simulink model "HANcoder_E407_GTSync_v4"  (R2018b)
settings: Solver=FixedStepDiscrete  StartTime=0.0  StopTime=1  FixedStep=0.01  RelTol=1e-3
PreLoadFcn:
  | librarySetup
  | eval([bdroot,'_startup']) %Calling [modelName]_startup.m
values from neighbouring files (symbols this model uses):
  basic_cycle_duration = TM12 + COMP_duration    (= 495)    [HANcoder_E407_GTSync_v4_startup.m]
  COM_Period = 100    [HANcoder_E407_GTSync_v4_startup.m]
  COM_Phase = COM_Period/2    (= 50)    [HANcoder_E407_GTSync_v4_startup.m]
  comm_delay_estimation = 20    [HANcoder_E407_GTSync_v4_startup.m]
  frequency_IRQ = 20    [HANcoder_E407_GTSync_v4_startup.m]
  HANtuneOverride = Simulink.Parameter    [HANcoder_E407_GTSync_v4_startup.m]
  idle_time_init = basic_cycle_duration*matrix_rows    (= 990)    [HANcoder_E407_GTSync_v4_startup.m]
  LED_ticks_toggle = 10000    [HANcoder_E407_GTSync_v4_startup.m]
  Master_Role = 1    [HANcoder_E407_GTSync_v4_startup.m]
  matrix_rows = 2    [HANcoder_E407_GTSync_v4_startup.m]
  Slave_Role = 2    [HANcoder_E407_GTSync_v4_startup.m]
  Sync_ID = 1    [HANcoder_E407_GTSync_v4_startup.m]
  time_difference_threshold = 500    [HANcoder_E407_GTSync_v4_startup.m]
  TM0 = basic_cycle_start    (= 5)    [HANcoder_E407_GTSync_v4_startup.m]
  TM1 = TM0 + COMM_duration    (= 105)    [HANcoder_E407_GTSync_v4_startup.m]
  TM10 = TM9  + COMP_duration    (= 465)    [HANcoder_E407_GTSync_v4_startup.m]
  TM11 = TM10 + COMP_duration    (= 475)    [HANcoder_E407_GTSync_v4_startup.m]
  TM12 = TM11 + COMP_duration    (= 485)    [HANcoder_E407_GTSync_v4_startup.m]
  TM2 = TM1 + COMP_duration    (= 115)    [HANcoder_E407_GTSync_v4_startup.m]
  TM3 = TM2 + COMP_duration    (= 125)    [HANcoder_E407_GTSync_v4_startup.m]
  TM4 = TM3 + COMM_duration    (= 225)    [HANcoder_E407_GTSync_v4_startup.m]
  TM5 = TM4 + COMP_duration    (= 235)    [HANcoder_E407_GTSync_v4_startup.m]
  TM6 = TM5 + COMM_duration    (= 335)    [HANcoder_E407_GTSync_v4_startup.m]
  TM7 = TM6 + COMP_duration    (= 345)    [HANcoder_E407_GTSync_v4_startup.m]
  TM8 = TM7 + COMM_duration    (= 445)    [HANcoder_E407_GTSync_v4_startup.m]
  TM9 = TM8  + COMP_duration    (= 455)    [HANcoder_E407_GTSync_v4_startup.m]
  Vote1_ID = 12    [HANcoder_E407_GTSync_v4_startup.m]
  Vote2_ID = 22    [HANcoder_E407_GTSync_v4_startup.m]
  Vote3_ID = 32    [HANcoder_E407_GTSync_v4_startup.m]
  wrap_up_threshold = basic_cycle_duration - time_difference_threshold*10    (= -4505)    [HANcoder_E407_GTSync_v4_startup.m]
undefined symbols (not defined in the file or in its folder): A0, A1, CON2
libraries: HANcoder_STM32_Target x22, simulink x3, hdlsllib x2, simulink_extras x1
(part 5 of 5)

== system HANcoder_E407_GTSync_v4/HANcoder STM32 Target - E407-STM32 algorithm/Global Ticks Increment/CAN Management/Matrix Cycle Manager/COMP Task - Update LT1/Local Time Update/Process Time Difference/Check_Wrap_up1 ==
  In1 : Inport
  GreaterThan : RelationalOperator  Operator=>  OutDataTypeStr=boolean  RndMeth=Simplest
  Minus : Sum  Inputs=+-
  Switch : Switch  Criteria=u2 > Threshold
  Wrap-up_Threshold : Constant  Value=wrap_up_threshold
  Wrap-up_Threshold1 : Constant  Value=basic_cycle_duration
  Out1 : Outport
  wires:
  In1/1 -> Minus/1, Switch/3, GreaterThan/1
  Wrap-up_Threshold/1 -> GreaterThan/2
  GreaterThan/1 -> Switch/2
  Switch/1 -> Out1/1
  Minus/1 -> Switch/1
  Wrap-up_Threshold1/1 -> Minus/2

== stateflow chart HANcoder_E407_GTSync_v4/HANcoder STM32 Target - E407-STM32 algorithm/Global Ticks Increment/Function-Call Subsystem/Even_Tick ==
  settings: initializeOutput=1
  state Even_tick
    if (mod(current_tick,2)==0)
    active_flag = 1;
    end
  state Rise_edge
    send(rise_edge_at_even)
  (default) -> Even_tick
  Even_tick -> Rise_edge : [active_flag == 1]
  data: current_tick input; active_flag local =0
  events: rise_edge_at_even output EITHER_EDGE_EVENT

== stateflow chart HANcoder_E407_GTSync_v4/HANcoder STM32 Target - E407-STM32 algorithm/Global Ticks Increment/Function-Call Subsystem/Chart ==
  state Send_Trigger
    if (Condition)
    send(Trigger_Signal)
    end
  (default) -> Send_Trigger
  data: Condition input
  events: Trigger_Signal output FUNCTION_CALL_EVENT

== stateflow chart HANcoder_E407_GTSync_v4/HANcoder STM32 Target - E407-STM32 algorithm/Global Ticks Increment/Function-Call Subsystem/Odd_Tick ==
  settings: initializeOutput=1
  state Odd_tick
    if (mod(current_tick,2)==1)
    active_flag = 1;
    end
  state Rise_edge
    send(rise_edge_at_odd)
  (default) -> Odd_tick
  Odd_tick -> Rise_edge : [active_flag == 1]
  data: current_tick input; active_flag local =0
  events: rise_edge_at_odd output EITHER_EDGE_EVENT

== stateflow chart HANcoder_E407_GTSync_v4/HANcoder STM32 Target - E407-STM32 algorithm/Global Ticks Increment/CAN Management/Chart ==
  state Send_Trigger
    if (Condition)
    send(Trigger_Signal)
    end
  (default) -> Send_Trigger
  data: Condition input
  events: Trigger_Signal output FUNCTION_CALL_EVENT

== stateflow chart HANcoder_E407_GTSync_v4/HANcoder STM32 Target - E407-STM32 algorithm/Global Ticks Increment/CAN Management/Chart1 ==
  state Send_Trigger
    if (Condition)
    send(Trigger_Signal)
    end
  (default) -> Send_Trigger
  data: Condition input
  events: Trigger_Signal output FUNCTION_CALL_EVENT
